simulink model "buck_conv_current"  (R2015a)
settings: Solver=ode45  StartTime=0.0  StopTime=0.001  FixedStep=1e-6  RelTol=1e-3
libraries: powerlib x9, powerlib_meascontrol x1
settings Model: Creator=ROHITH  LastModifiedBy=ROHITH
settings DebuggingCC: MaxConsecutiveZCsMsg=none

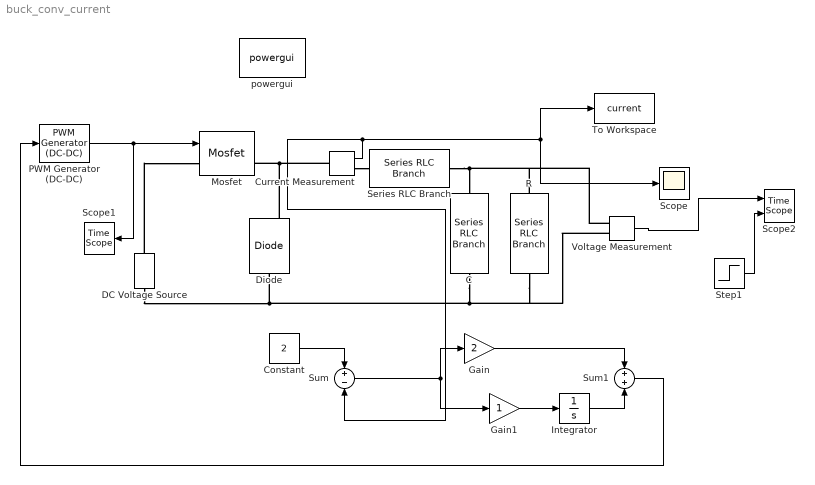
== system buck_conv_current ==
  C : powerlib/Elements/Series RLC Branch  LConnTagsString=__new0  RConnTagsString=__new0  BranchType=C  Resistance=1  Inductance=1e-3  SetiL0=off  InitialCurrent=0  Capacitance=2e-5  Setx0=off  InitialVoltage=0  Measurements=None
  Constant : Constant  Value=2
  Current Measurement : powerlib/Measurements/Current Measurement  PhasorSimulation=off  OutputType=Complex  PSBequivalent=0
  DC Voltage Source : powerlib/Electrical Sources/DC Voltage Source  Amplitude=12  Measurements=None
  Diode : powerlib/Power Electronics/Diode  Ron=0.001  Lon=0  Vf=0.8  IC=0  UseSnubber=off  Rs=500  Cs=250e-9  Measurements=on
  Gain : Gain  Gain=2
  Gain1 : Gain
  Integrator : Integrator
  Mosfet : powerlib/Power Electronics/Mosfet  Ron=0.1  Lon=0  Rd=0.01  Vfd=0  IC=0  Rs=1e5  Cs=inf  Measurements=on
  PWM Generator (DC-DC) : powerlib_meascontrol/Pulse & Signal Generators/PWM Generator (DC-DC)  Fsw=100000  Ts=0
  R : powerlib/Elements/Series RLC Branch  LConnTagsString=__new0  RConnTagsString=__new0  BranchType=R  Resistance=1.25  Inductance=1e-3  SetiL0=off  InitialCurrent=0  Capacitance=1e-6  Setx0=off  InitialVoltage=0  Measurements=None
  Scope : Scope
      settings: SaveName=ScopeData2
  Scope1 : TimeScope
  Scope2 : TimeScope  NumInputPorts=2
  Series RLC Branch : powerlib/Elements/Series RLC Branch  LConnTagsString=__new0  RConnTagsString=__new0  BranchType=L  Resistance=1  Inductance=3.64e-5  SetiL0=off  InitialCurrent=0  Capacitance=1e-6  Setx0=off  InitialVoltage=0  Measurements=None
  Step1 : Step  Time=0.005  Before=5  After=3  SampleTime=0
  Sum : Sum  Inputs=+-
  Sum1 : Sum
  To Workspace : ToWorkspace  VariableName=current  SaveFormat=Timeseries  SampleTime=-1
  Voltage Measurement : powerlib/Measurements/Voltage Measurement  PhasorSimulation=off  OutputType=Complex  PSBequivalent=0
  powergui : powerlib/powergui  Priority=1  SimulationMode=Continuous  SolverType=Tustin/Backward Euler (TBE)  SampleTime=50e-6  frequency=60  SPID=off  DisableSnubberDevices=off  DisableRonSwitches=off  DisableVfSwitches=off  SwTol=0  DisplayEquations=off  Interpol=off  methode=off  Ts=100  FunctionMessages=off  echomessages=off  HookPort=off  EnableUseOfTLC=off  x0status=blocks  frequencyindice=0  Pbase=100e6  ErrMax=1e-4  Iterations=50  UnitsV=kV  UnitsW=MW  buscounter=0  RestoreLinks=warning  ResistiveCurrentMeasurement=off  Frange=[0:2:500]  Ylog=off  Xlog=on  ShowGrid=off  save=off  variable=ZData  structure=0  ZoomFFT=off  StartTime=0.0  cycles=1  DisplayStyle=1  fundamental=60  FreqAxis=off  MaxFrequency=1000  frequencyindicesteady=1  RmsSteady=1  display=off
  wires:
  Voltage Measurement/1 -> Scope2/1
  Current Measurement/1 -> To Workspace/1, Scope/1, Sum/2
  PWM Generator (DC-DC)/1 -> Scope1/1, Mosfet/1
  Step1/1 -> Scope2/2
  Gain1/1 -> Integrator/1
  Sum/1 -> Gain1/1, Gain/1
  Gain/1 -> Sum1/1
  Integrator/1 -> Sum1/2
  Constant/1 -> Sum/1
  Sum1/1 -> PWM Generator (DC-DC)/1
  connections:
  DC Voltage Source/RConn1 -- Mosfet/LConn1
  Diode/RConn1 -- Mosfet/RConn1 -- Current Measurement/LConn1
  DC Voltage Source/LConn1 -- R/RConn1 -- Voltage Measurement/LConn2 -- C/LConn1 -- Diode/LConn1
  Series RLC Branch/RConn1 -- R/LConn1 -- Voltage Measurement/LConn1 -- C/RConn1
  Current Measurement/RConn1 -- Series RLC Branch/LConn1
